simulink model "Dc_Motor"  (R2023a)
settings: Solver=ode15s  StartTime=0.0  StopTime=10.0  RelTol=1e-3
model workspace (MAT data in the model file):
  J = 5e-05
  K = 0.2
  L = 0.01
  R = 4
  Sig = Simulink.Signal
  Sig.DataType = 'auto'
  Sig.Dimensions = -1
  Sig.DimensionsMode = 'auto'
  Sig.Complexity = 'auto'
  Sig.SampleTime = -1
  Sig.SamplingMode = 'auto'
  V = 7.4
  b = 0.0005
settings Model: Creator=MY PC  LastModifiedBy=MY PC

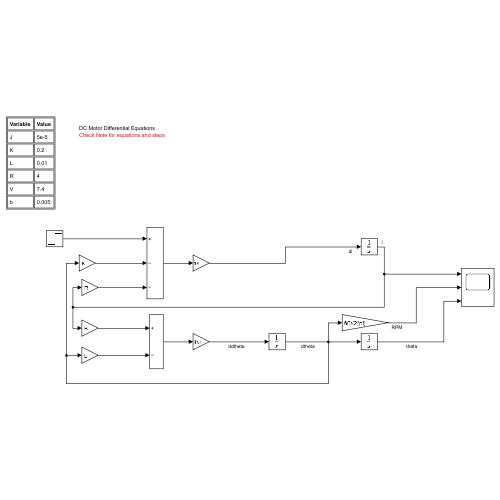
[thumbnail: Simulink's stored preview of the top-level diagram]
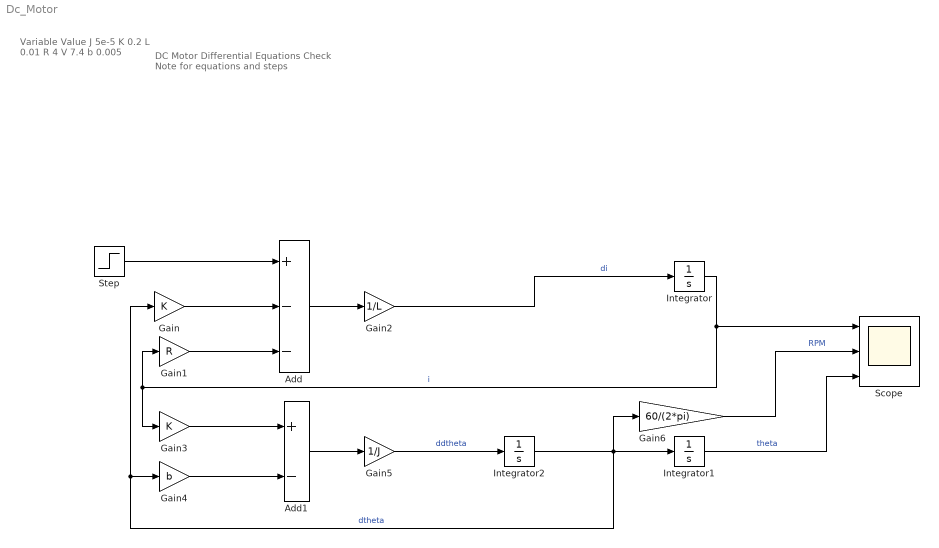
== system Dc_Motor ==
  note: DC Motor Differential Equations
      | Check Note for equations and steps
  note: Variable
      | Value
      |
      | J
      | 5e-5
      |
      | K
      | 0.2
      |
      | L
      | 0.01
      |
      | R
      | 4
      |
      | V
      | 7.4
      |
      | b
      | 0.005
  Add : Sum  Inputs=+--
  Add1 : Sum  Inputs=+-
  Gain : Gain  Gain=K
  Gain1 : Gain  Gain=R
  Gain2 : Gain  Gain=1/L
  Gain3 : Gain  Gain=K
  Gain4 : Gain  Gain=b
  Gain5 : Gain  Gain=1/J
  Gain6 : Gain  Gain=60/(2*pi)
  Integrator : Integrator
  Integrator1 : Integrator
  Integrator2 : Integrator
  Scope : Scope  NumInputPorts=3
  Step : Step  After=V  SampleTime=0
  wires:
  Gain2/1 -> Integrator/1  "di"
  Integrator/1 -> Scope/1, Gain1/1, Gain3/1  "i"
  Integrator1/1 -> Scope/3  "theta"
  Integrator2/1 -> Gain6/1, Gain4/1, Gain/1, Integrator1/1  "dtheta"
  Gain5/1 -> Integrator2/1  "ddtheta"
  Step/1 -> Add/1
  Gain/1 -> Add/2
  Gain1/1 -> Add/3
  Add/1 -> Gain2/1
  Gain3/1 -> Add1/1
  Gain4/1 -> Add1/2
  Add1/1 -> Gain5/1
  Gain6/1 -> Scope/2  "RPM"
